simulink library "thermochemical"  (R2017b)
settings: Solver=VariableStepAuto  StartTime=0.0  StopTime=10.0  RelTol=1e-3
values from neighbouring files (symbols this model uses):
  c = conversion_factors()    [blk_clausius_clapeyron.m]    (also in blk_clausius_clapeyron_no_popup.m; blk_cold_room_closed_dry_air.m; blk_reactor_BaCl2_NH3_no_walls.m; blk_reactor_BaCl2_NH3_no_walls_state_space.m)
  cp = metal.cp    [blk_wall_simple.m]    (also in get_metal_properties.m = 390)
  fluid = get_param(blk,'fluid')    [blk_thermodynamic_properties_nonsaturated.m]    (also in blk_thermodynamic_properties_nonsaturated_interpreted.m; blk_thermodynamic_properties_saturated.m; blk_thermodynamic_properties_saturated_interpreted.m; blk_thermodynamic_properties_saturated_mix.m)
  gas = get_material_properties(x.gasName)    [blk_reactor_BaCl2_NH3_cylindrical_no_walls_fun1.m]
  h = get_param(gcb,'ObjectParameters')    [get_param_eval.m]
  rho = metal.rho    [blk_wall_simple.m]    (also in get_metal_properties.m = 8940)
  s = solve(eq,dx,'ReturnConditions',true)    [LMTD_inv.m]    (also in blk_wall_simple.m = get_param_eval(blk,'s'))
  u_gas_at_T_ref = -R * T_ref    [blk_reactor_BaCl2_NH3_no_walls.m]    (also in blk_reactor_BaCl2_NH3_no_walls_state_space.m)
undefined symbols (not defined in the file or in its folder): b_motor, BaCl2, beta, CoolProp, cP_binder, cP_gas, cP_s0, cv, dh_r_0, ENG, heat_exchanger_epsilonNTU_inv_simulink, heat_exchanger_epsilonNTU_simulink, J_motor, K_cin, kappa, Km_motor, La_motor, lookup2D_BreakPoint2, M_binder, N_binder, N_gas_free_volume_init, N_salt, NH3, nh3_v3, nu, P, phase, PID_D_motor, PID_I_motor, PID_P_motor, Ra_motor, Reactor_phase, T, T1, T2, T_init, Tr_init, Tr_ref, U_binder_at_Tr_ref, U_salt_at_X0_Tr_ref, Ur_init, V_void, Valve_regime, Vmax_motor, w_init_motor, X_init
libraries: thermochemical x247, simulink x54, dspsigops x3
(part 4 of 12)

== system thermochemical/Reactors/Reactor, BaCl2//NH3, state-space form, [Tr, Ng, X] as state variables, no algebraic loops, ideal gas in void volume, ideal gas in salt ==
  "Reactor, BaCl2, cylindrical, finned tube, state-space form, [Tr, Ng, X] as state variables, no algebraic loops, ideal gas in void volume" : Subsystem
  "Reactor, BaCl2/NH3, cylindrical, no walls, state-space form, [Tr, Ng, X] as state variables, no algebraic loops, ideal gas in void volume" : Subsystem  LoadFcn=Simulink.defineIntEnumType('Reactor_phase',{'Synthesis','No_reaction','Desorption'},[1 0 -1])  mask(reactor_BaCl2_NH3_cylindrical_no_walls){pairName=Barium chloride/Ammonia (BaCl2/NH3), gasName=Ammonia gas (NH3), binderName=ENG, tao_salt=0.75, rho_composite=300, K_cin=1e-3, fluid=nh3_v3, Lr=1.5, Lr_total=1.6, Dr=0.11, Ddiff=0.018, Tr_init=300, X_init=0.1, Vr_L=15.2053, m_composite_kg=4.162, m_salt_kg=3.1215, m_binder_kg=1.0405, m_gas_when_reactor_fully_charged_kg=2.0423, kWh_cold=0.77838, N_salt=14.9906, N_binder=86.6307, V_void=0.001332, N_gas_free_volume_init=0.16063}
      mask prompts: pairName "Pair name"; gasName "Gas name"; binderName "Binder name"; tao_salt "Salt/Composite mass ratio (mass salt/mass mixture)"; rho_composite "Composite density (kg/m3 of composite)"; K_cin "Reaction's rate constant [1/sec]"; fluid "Gas look-up table data (structure variable):"; Lr "Reactor effective length (section filled with composite) [m]"; Lr_total "Reactor total length ( > effective length) [m]"; Dr "Reactor diameter [m]"; Ddiff "Central diffuser diameter [m]"; Tr_init "Reactor initial temperature [K]"; X_init "Reaction's advancement initial state X0 [0..1]"; Vr_L "Volume reactor (litre)"; m_composite_kg "Mass of composite (salt + binder) (kg)"; m_salt_kg "Mass of salt (kg)"; m_binder_kg "Mass of binder (kg)"; m_gas_when_reactor_fully_charged_kg "Mass of gas (when reactor is fully charged) (kg)"; kWh_cold "Estimated cold production during synthesis (kWh)"; N_salt "Number of mols of salt [mol]"; N_binder "Number of mols of binder [mol]"; V_void "Reactor void volume [m3]"; N_gas_free_volume_init "Initial number of mols of gas in the reactor's free volume [mol]"
      mask help:
      | Solid/Gas thermochemical reactor model, cylindrical shape (no walls)
      | Pair: Barium chloride/Ammonia (BaCl2/NH3)
      mask init:
      | % Note: the enumerated type is declared in 
      | % the 'LoadFnc' callback of the block. In cannot be 
      | % declared here because it gives error for duplicate
      | % declaration.
      | blk_reactor_BaCl2_NH3_cylindrical_no_walls(gcb)
      mask DialogControl Container21 Prompt: Input parameters
      mask DialogControl Container34 Prompt: Reactor's parameters
      mask DialogControl Container31 Prompt: Geometry
      mask DialogControl Container33 Prompt: Reactor Initial state
      mask DialogControl Container18 Prompt: Info (read-only)
      mask DialogControl Container16 Prompt: Base block inputs (read-only)
  "Reactor, BaCl2/NH3, no walls, state-space form, [Tr, Ng, X] as state variables, no algebraic loops, ideal gas in void volume" : Subsystem  LoadFcn=Simulink.defineIntEnumType('Reactor_phase',{'Synthesis','No_reaction','Desorption'},[1 0 -1])  mask(reactor_BaCl2_NH3_no_walls_state_space){pairName=Barium chloride/Ammonia (BaCl2/NH3), gasName=Ammonia gas (NH3), binderName=ENG, N_salt=N_salt, N_binder=N_binder, K_cin=K_cin, V_void=V_void, fluid=fluid, Tr_init=Tr_init, X_init=X_init, N_gas_free_volume_init=N_gas_free_volume_init, m_composite_kg=3.223, m_salt_kg=2.385, m_binder_kg=0.83797, m_gas_when_reactor_fully_charged=1.5605, T_ref=300, u_gas_at_T_ref=0, U_binder_at_T_ref=0, U_salt_at_X0_T_ref=0, R=8.3145, cP_gas=42.5775, cV_gas=29.4370, nu=8, cP_s0=75.1, dh_r_0=38250, M_binder=0.012011, cP_binder=714.36, P_dead_zone=0.0001, dn_dead_zone=0.0001}
      mask prompts: pairName "Pair name"; gasName "Gas name"; binderName "Binder name"; N_salt "Number of mols of salt [mol]"; N_binder "Number of mols of binder [mol]"; K_cin "Reaction's rate constant [1/sec]"; V_void "Reactor void volume [m3]"; fluid "Gas look-up table data (structure variable):"; Tr_init "Reactor initial temperature [K]"; X_init "Reaction's advancement initial state X0 [0..1]"; N_gas_free_volume_init "Initial number of mols of gas in the reactor's void volume [mol]"; m_composite_kg "Mass of composite (salt + binder) (kg)"; m_salt_kg "Mass of salt (kg)"; m_binder_kg "Mass of binder (kg)"; m_gas_when_reactor_fully_charged "Mass of gas (when reactor is fully charged) (kg)"; T_ref "Reference temperature of gas (for the internal energy equation) [K]"; u_gas_at_T_ref "Gas specific internal energy at reference temperature [J/mol]"; U_binder_at_T_ref "Binder internal energy at reference temperature [J]"; U_salt_at_X0_T_ref "Salt internal energy at X=0 and at reference temperature [J]"; R "Universal gas constant [J/K/mol]"; cP_gas "Cp of gas [J/K/mol]"; cV_gas "Cv of gas [J/K/mol]"; nu "Reaction stoichiometric coefficient [mol gas/mol salt]"; cP_s0 "Cp of the anhydrous salt [J/(K.mol)]"; dh_r_0 "Standard enthalpy of reaction [J/mol of gas]"; M_binder "Molar mass of binder [kg/mol]"; cP_binder "Cp of binder [J/(K.kg)]"; P_dead_zone "Presure hystesis to avoid chattering between adsorption and desorption models (typical value: 1e-4) [bar]"; dn_dead_zone "Flow rate hysteresis to avoid chattering between adsorption and desorption models (typical value: 1e-4) [mol/sec]"
      mask help:
      | Solid/Gas thermochemical reactor model (no walls)
      | Pair: Barium chloride/Ammonia (BaCl2/NH3)
      mask init:
      | % Note: the enumerated type is declared in 
      | % the 'LoadFnc' callback of the block. In cannot be 
      | % declared here because it gives error for duplicate
      | % declaration.
      | 
      | blk_reactor_BaCl2_NH3_no_walls_state_space(gcb)
      mask DialogControl Container21 Prompt: Input parameters
      mask DialogControl Container34 Prompt: Reactor's parameters
      mask DialogControl Container33 Prompt: Reactor Initial state
      mask DialogControl Container32 Prompt: Info (read-only)
      mask DialogControl Container16 Prompt: Other read-only parameters
      mask DialogControl Container20 Prompt: References
      mask DialogControl Container18 Prompt: Gas
      mask DialogControl Container47 Prompt: Solid/Gas
      mask DialogControl Container19 Prompt: Binder
      mask DialogControl Container26 Prompt: Other model's parameters

== system thermochemical/Reactors/Reactor, BaCl2//NH3, state-space form, [Tr, Ng, X] as state variables, no algebraic loops, real gas in void volume, ideal gas in salt ==
  "Reactor, BaCl2, cylindrical, finned tube, state-space form, [Tr, Ng, X] as state variables, no algebraic loops, real gas in void volume, ideal gas in salt" : Subsystem
  "Reactor, BaCl2/NH3, cylindrical, no walls, state-space form, [Tr, Ng, X] as state variables, no algebraic loops, real gas in void volume, ideal gas in salt" : Subsystem  LoadFcn=Simulink.defineIntEnumType('Reactor_phase',{'Synthesis','No_reaction','Desorption'},[1 0 -1])  mask(reactor_BaCl2_NH3_cylindrical_no_walls){pairName=Barium chloride/Ammonia (BaCl2/NH3), gasName=Ammonia gas (NH3), binderName=ENG, tao_salt=0.75, rho_composite=300, K_cin=1e-3, fluid=nh3_v3, Lr=1.5, Lr_total=1.6, Dr=0.11, Ddiff=0.018, Tr_init=300, X_init=0.1, Vr_L=15.2053, m_composite_kg=4.162, m_salt_kg=3.1215, m_binder_kg=1.0405, m_gas_when_reactor_fully_charged_kg=2.0423, kWh_cold=0.77838, N_salt=14.9906, N_binder=86.6307, V_void=0.001332, N_gas_free_volume_init=0.16063}
      mask prompts: pairName "Pair name"; gasName "Gas name"; binderName "Binder name"; tao_salt "Salt/Composite mass ratio (mass salt/mass mixture)"; rho_composite "Composite density (kg/m3 of composite)"; K_cin "Reaction's rate constant [1/sec]"; fluid "Gas look-up table data (structure variable):"; Lr "Reactor effective length (section filled with composite) [m]"; Lr_total "Reactor total length ( > effective length) [m]"; Dr "Reactor diameter [m]"; Ddiff "Central diffuser diameter [m]"; Tr_init "Reactor initial temperature [K]"; X_init "Reaction's advancement initial state X0 [0..1]"; Vr_L "Volume reactor (litre)"; m_composite_kg "Mass of composite (salt + binder) (kg)"; m_salt_kg "Mass of salt (kg)"; m_binder_kg "Mass of binder (kg)"; m_gas_when_reactor_fully_charged_kg "Mass of gas (when reactor is fully charged) (kg)"; kWh_cold "Estimated cold production during synthesis (kWh)"; N_salt "Number of mols of salt [mol]"; N_binder "Number of mols of binder [mol]"; V_void "Reactor void volume [m3]"; N_gas_free_volume_init "Initial number of mols of gas in the reactor's free volume [mol]"
      mask help:
      | Solid/Gas thermochemical reactor model, cylindrical shape (no walls)
      | Pair: Barium chloride/Ammonia (BaCl2/NH3)
      mask init: same as thermochemical/Reactors/Reactor, BaCl2//NH3, state-space form, [Tr, Ng, X] as state variables, no algebraic loops, ideal gas in void volume, ideal gas in salt/Reactor, BaCl2/NH3, cylindrical, no walls, state-space form, [Tr, Ng, X] as state variables, no algebraic loops, ideal gas in void volume
      mask DialogControl Container21 Prompt: Input parameters
      mask DialogControl Container34 Prompt: Reactor's parameters
      mask DialogControl Container31 Prompt: Geometry
      mask DialogControl Container33 Prompt: Reactor Initial state
      mask DialogControl Container18 Prompt: Info (read-only)
      mask DialogControl Container16 Prompt: Base block inputs (read-only)
  "Reactor, BaCl2/NH3, no walls, state-space form, [Tr, Ng, X] as state variables, no algebraic loops, real gas in void volume, ideal gas in salt" : Subsystem  LoadFcn=Simulink.defineIntEnumType('Reactor_phase',{'Synthesis','No_reaction','Desorption'},[1 0 -1])  mask(reactor_BaCl2_NH3_no_walls_state_space){pairName=Barium chloride/Ammonia (BaCl2/NH3), gasName=Ammonia gas (NH3), binderName=ENG, N_salt=N_salt, N_binder=N_binder, K_cin=K_cin, V_void=V_void, fluid=fluid, Tr_init=Tr_init, X_init=X_init, N_gas_free_volume_init=N_gas_free_volume_init, m_composite_kg=3.223, m_salt_kg=2.385, m_binder_kg=0.83797, m_gas_when_reactor_fully_charged=1.5605, T_ref=300, u_gas_at_T_ref=0, U_binder_at_T_ref=0, U_salt_at_X0_T_ref=0, R=8.3145, cP_gas=42.5775, cV_gas=29.4370, nu=8, cP_s0=75.1, dh_r_0=38250, M_binder=0.012011, cP_binder=714.36, P_dead_zone=0.0001, dn_dead_zone=0.0001}
      mask prompts: pairName "Pair name"; gasName "Gas name"; binderName "Binder name"; N_salt "Number of mols of salt [mol]"; N_binder "Number of mols of binder [mol]"; K_cin "Reaction's rate constant [1/sec]"; V_void "Reactor void volume [m3]"; fluid "Gas look-up table data (structure variable):"; Tr_init "Reactor initial temperature [K]"; X_init "Reaction's advancement initial state X0 [0..1]"; N_gas_free_volume_init "Initial number of mols of gas in the reactor's void volume [mol]"; m_composite_kg "Mass of composite (salt + binder) (kg)"; m_salt_kg "Mass of salt (kg)"; m_binder_kg "Mass of binder (kg)"; m_gas_when_reactor_fully_charged "Mass of gas (when reactor is fully charged) (kg)"; T_ref "Reference temperature of gas (for the internal energy equation) [K]"; u_gas_at_T_ref "Gas specific internal energy at reference temperature [J/mol]"; U_binder_at_T_ref "Binder internal energy at reference temperature [J]"; U_salt_at_X0_T_ref "Salt internal energy at X=0 and at reference temperature [J]"; R "Universal gas constant [J/K/mol]"; cP_gas "Cp of gas [J/K/mol]"; cV_gas "Cv of gas [J/K/mol]"; nu "Reaction stoichiometric coefficient [mol gas/mol salt]"; cP_s0 "Cp of the anhydrous salt [J/(K.mol)]"; dh_r_0 "Standard enthalpy of reaction [J/mol of gas]"; M_binder "Molar mass of binder [kg/mol]"; cP_binder "Cp of binder [J/(K.kg)]"; P_dead_zone "Presure hystesis to avoid chattering between adsorption and desorption models (typical value: 1e-4) [bar]"; dn_dead_zone "Flow rate hysteresis to avoid chattering between adsorption and desorption models (typical value: 1e-4) [mol/sec]"
      mask help:
      | Solid/Gas thermochemical reactor model (no walls)
      | Pair: Barium chloride/Ammonia (BaCl2/NH3)
      mask init: same as thermochemical/Reactors/Reactor, BaCl2//NH3, state-space form, [Tr, Ng, X] as state variables, no algebraic loops, ideal gas in void volume, ideal gas in salt/Reactor, BaCl2/NH3, no walls, state-space form, [Tr, Ng, X] as state variables, no algebraic loops, ideal gas in void volume
      mask DialogControl Container21 Prompt: Input parameters
      mask DialogControl Container34 Prompt: Reactor's parameters
      mask DialogControl Container33 Prompt: Reactor Initial state
      mask DialogControl Container32 Prompt: Info (read-only)
      mask DialogControl Container16 Prompt: Other read-only parameters
      mask DialogControl Container20 Prompt: References
      mask DialogControl Container18 Prompt: Gas
      mask DialogControl Container47 Prompt: Solid/Gas
      mask DialogControl Container19 Prompt: Binder
      mask DialogControl Container26 Prompt: Other model's parameters

== system thermochemical/Reactors/Reactor, BaCl2//NH3, state-space form, [Tr, Ng, X] as state variables, no algebraic loops, real gas in void volume, real gas in salt ==
  "Reactor, BaCl2, cylindrical, finned tube, state-space form, [Tr, Ng, X] as state variables, no algebraic loops, real gas in void volume, real gas in salt" : Subsystem
  "Reactor, BaCl2/NH3, cylindrical, no walls, state-space form, [Tr, Ng, X] as state variables, no algebraic loops, real gas in void volume, real gas in salt" : Subsystem  LoadFcn=Simulink.defineIntEnumType('Reactor_phase',{'Synthesis','No_reaction','Desorption'},[1 0 -1])  mask(reactor_BaCl2_NH3_cylindrical_no_walls){pairName=Barium chloride/Ammonia (BaCl2/NH3), gasName=Ammonia gas (NH3), binderName=ENG, tao_salt=0.75, rho_composite=300, K_cin=1e-3, fluid=nh3_v3, Lr=1.5, Lr_total=1.6, Dr=0.11, Ddiff=0.018, Tr_init=300, X_init=0.1, Vr_L=15.2053, m_composite_kg=4.162, m_salt_kg=3.1215, m_binder_kg=1.0405, m_gas_when_reactor_fully_charged_kg=2.0423, kWh_cold=0.77838, N_salt=14.9906, N_binder=86.6307, V_void=0.001332, N_gas_free_volume_init=0.16063}
      mask prompts: pairName "Pair name"; gasName "Gas name"; binderName "Binder name"; tao_salt "Salt/Composite mass ratio (mass salt/mass mixture)"; rho_composite "Composite density (kg/m3 of composite)"; K_cin "Reaction's rate constant [1/sec]"; fluid "Gas look-up table data (structure variable):"; Lr "Reactor effective length (section filled with composite) [m]"; Lr_total "Reactor total length ( > effective length) [m]"; Dr "Reactor diameter [m]"; Ddiff "Central diffuser diameter [m]"; Tr_init "Reactor initial temperature [K]"; X_init "Reaction's advancement initial state X0 [0..1]"; Vr_L "Volume reactor (litre)"; m_composite_kg "Mass of composite (salt + binder) (kg)"; m_salt_kg "Mass of salt (kg)"; m_binder_kg "Mass of binder (kg)"; m_gas_when_reactor_fully_charged_kg "Mass of gas (when reactor is fully charged) (kg)"; kWh_cold "Estimated cold production during synthesis (kWh)"; N_salt "Number of mols of salt [mol]"; N_binder "Number of mols of binder [mol]"; V_void "Reactor void volume [m3]"; N_gas_free_volume_init "Initial number of mols of gas in the reactor's free volume [mol]"
      mask help:
      | Solid/Gas thermochemical reactor model, cylindrical shape (no walls)
      | Pair: Barium chloride/Ammonia (BaCl2/NH3)
      mask init: same as thermochemical/Reactors/Reactor, BaCl2//NH3, state-space form, [Tr, Ng, X] as state variables, no algebraic loops, ideal gas in void volume, ideal gas in salt/Reactor, BaCl2/NH3, cylindrical, no walls, state-space form, [Tr, Ng, X] as state variables, no algebraic loops, ideal gas in void volume
      mask DialogControl Container21 Prompt: Input parameters
      mask DialogControl Container34 Prompt: Reactor's parameters
      mask DialogControl Container31 Prompt: Geometry
      mask DialogControl Container33 Prompt: Reactor Initial state
      mask DialogControl Container18 Prompt: Info (read-only)
      mask DialogControl Container16 Prompt: Base block inputs (read-only)
  "Reactor, BaCl2/NH3, no walls, state-space form, [Tr, Ng, X] as state variables, no algebraic loops, real gas in void volume, real gas in salt" : Subsystem  LoadFcn=Simulink.defineIntEnumType('Reactor_phase',{'Synthesis','No_reaction','Desorption'},[1 0 -1])  mask(reactor_BaCl2_NH3_no_walls_state_space){pairName=Barium chloride/Ammonia (BaCl2/NH3), gasName=Ammonia gas (NH3), binderName=ENG, N_salt=N_salt, N_binder=N_binder, K_cin=K_cin, V_void=V_void, fluid=fluid, Tr_init=Tr_init, X_init=X_init, N_gas_free_volume_init=N_gas_free_volume_init, m_composite_kg=3.223, m_salt_kg=2.385, m_binder_kg=0.83797, m_gas_when_reactor_fully_charged=1.5605, T_ref=300, u_gas_at_T_ref=0, U_binder_at_T_ref=0, U_salt_at_X0_T_ref=0, R=8.3145, cP_gas=42.5775, cV_gas=29.4370, nu=8, cP_s0=75.1, dh_r_0=38250, M_binder=0.012011, cP_binder=714.36, P_dead_zone=0.0001, dn_dead_zone=0.0001}
      mask prompts: pairName "Pair name"; gasName "Gas name"; binderName "Binder name"; N_salt "Number of mols of salt [mol]"; N_binder "Number of mols of binder [mol]"; K_cin "Reaction's rate constant [1/sec]"; V_void "Reactor void volume [m3]"; fluid "Gas look-up table data (structure variable):"; Tr_init "Reactor initial temperature [K]"; X_init "Reaction's advancement initial state X0 [0..1]"; N_gas_free_volume_init "Initial number of mols of gas in the reactor's void volume [mol]"; m_composite_kg "Mass of composite (salt + binder) (kg)"; m_salt_kg "Mass of salt (kg)"; m_binder_kg "Mass of binder (kg)"; m_gas_when_reactor_fully_charged "Mass of gas (when reactor is fully charged) (kg)"; T_ref "Reference temperature of gas (for the internal energy equation) [K]"; u_gas_at_T_ref "Gas specific internal energy at reference temperature [J/mol]"; U_binder_at_T_ref "Binder internal energy at reference temperature [J]"; U_salt_at_X0_T_ref "Salt internal energy at X=0 and at reference temperature [J]"; R "Universal gas constant [J/K/mol]"; cP_gas "Cp of gas [J/K/mol]"; cV_gas "Cv of gas [J/K/mol]"; nu "Reaction stoichiometric coefficient [mol gas/mol salt]"; cP_s0 "Cp of the anhydrous salt [J/(K.mol)]"; dh_r_0 "Standard enthalpy of reaction [J/mol of gas]"; M_binder "Molar mass of binder [kg/mol]"; cP_binder "Cp of binder [J/(K.kg)]"; P_dead_zone "Presure hystesis to avoid chattering between adsorption and desorption models (typical value: 1e-4) [bar]"; dn_dead_zone "Flow rate hysteresis to avoid chattering between adsorption and desorption models (typical value: 1e-4) [mol/sec]"
      mask help:
      | Solid/Gas thermochemical reactor model (no walls)
      | Pair: Barium chloride/Ammonia (BaCl2/NH3)
      mask init: same as thermochemical/Reactors/Reactor, BaCl2//NH3, state-space form, [Tr, Ng, X] as state variables, no algebraic loops, ideal gas in void volume, ideal gas in salt/Reactor, BaCl2/NH3, no walls, state-space form, [Tr, Ng, X] as state variables, no algebraic loops, ideal gas in void volume
      mask DialogControl Container21 Prompt: Input parameters
      mask DialogControl Container34 Prompt: Reactor's parameters
      mask DialogControl Container33 Prompt: Reactor Initial state
      mask DialogControl Container32 Prompt: Info (read-only)
      mask DialogControl Container16 Prompt: Other read-only parameters
      mask DialogControl Container20 Prompt: References
      mask DialogControl Container18 Prompt: Gas
      mask DialogControl Container47 Prompt: Solid/Gas
      mask DialogControl Container19 Prompt: Binder
      mask DialogControl Container26 Prompt: Other model's parameters

== system thermochemical/Reactors/Reactor, BaCl2//NH3, state-space form, [Ur, Ng, X] as state variables, no algebraic loops, ideal gas in void volume, ideal gas in salt ==
  "Reactor, BaCl2, cylindrical, finned tube, state-space form, [Ur, Ng, X] as state variables, no algebraic loops, ideal gas in void volume, ideal gas in salt" : Subsystem
  "Reactor, BaCl2/NH3, cylindrical, no walls, state-space form, [Ur, Ng, X] as state variables, no algebraic loops, ideal gas in void volume, ideal gas in salt" : Subsystem  LoadFcn=Simulink.defineIntEnumType('Reactor_phase',{'Synthesis','No_reaction','Desorption'},[1 0 -1])  mask(reactor_BaCl2_NH3_cylindrical_no_walls){pairName=Barium chloride/Ammonia (BaCl2/NH3), gasName=Ammonia gas (NH3), binderName=ENG, tao_salt=0.75, rho_composite=300, K_cin=1e-3, fluid=nh3_v3, Lr=1.5, Lr_total=1.6, Dr=0.11, Ddiff=0.018, Tr_init=300, X_init=0.1, Vr_L=15.2053, m_composite_kg=4.162, m_salt_kg=3.1215, m_binder_kg=1.0405, m_gas_when_reactor_fully_charged_kg=2.0423, kWh_cold=0.77838, N_salt=14.9906, N_binder=86.6307, V_void=0.001332, N_gas_free_volume_init=0.16063}
      mask prompts: pairName "Pair name"; gasName "Gas name"; binderName "Binder name"; tao_salt "Salt/Composite mass ratio (mass salt/mass mixture)"; rho_composite "Composite density (kg/m3 of composite)"; K_cin "Reaction's rate constant [1/sec]"; fluid "Gas look-up table data (structure variable):"; Lr "Reactor effective length (section filled with composite) [m]"; Lr_total "Reactor total length ( > effective length) [m]"; Dr "Reactor diameter [m]"; Ddiff "Central diffuser diameter [m]"; Tr_init "Reactor initial temperature [K]"; X_init "Reaction's advancement initial state X0 [0..1]"; Vr_L "Volume reactor (litre)"; m_composite_kg "Mass of composite (salt + binder) (kg)"; m_salt_kg "Mass of salt (kg)"; m_binder_kg "Mass of binder (kg)"; m_gas_when_reactor_fully_charged_kg "Mass of gas (when reactor is fully charged) (kg)"; kWh_cold "Estimated cold production during synthesis (kWh)"; N_salt "Number of mols of salt [mol]"; N_binder "Number of mols of binder [mol]"; V_void "Reactor void volume [m3]"; N_gas_free_volume_init "Initial number of mols of gas in the reactor's free volume [mol]"
      mask help:
      | Solid/Gas thermochemical reactor model, cylindrical shape (no walls)
      | Pair: Barium chloride/Ammonia (BaCl2/NH3)
      mask init: same as thermochemical/Reactors/Reactor, BaCl2//NH3, state-space form, [Tr, Ng, X] as state variables, no algebraic loops, ideal gas in void volume, ideal gas in salt/Reactor, BaCl2/NH3, cylindrical, no walls, state-space form, [Tr, Ng, X] as state variables, no algebraic loops, ideal gas in void volume
      mask DialogControl Container21 Prompt: Input parameters
      mask DialogControl Container34 Prompt: Reactor's parameters
      mask DialogControl Container31 Prompt: Geometry
      mask DialogControl Container33 Prompt: Reactor Initial state
      mask DialogControl Container18 Prompt: Info (read-only)
      mask DialogControl Container16 Prompt: Base block inputs (read-only)
  "Reactor, BaCl2/NH3, no walls, state-space form, [Ur, Ng, X] as state variables, no algebraic loops, ideal gas in void volume, ideal gas in salt" : Subsystem  LoadFcn=Simulink.defineIntEnumType('Reactor_phase',{'Synthesis','No_reaction','Desorption'},[1 0 -1])  mask(reactor_BaCl2_NH3_no_walls_state_space){pairName=Barium chloride/Ammonia (BaCl2/NH3), gasName=Ammonia gas (NH3), binderName=ENG, N_salt=N_salt, N_binder=N_binder, K_cin=K_cin, V_void=V_void, Tr_init=Tr_init, X_init=X_init, N_gas_free_volume_init=N_gas_free_volume_init, m_composite_kg=4.1639, m_salt_kg=3.1235, m_binder_kg=1.0405, m_gas_when_reactor_fully_charged=2.0436, T_ref=300, u_gas_at_T_ref=0, U_binder_at_T_ref=0, U_salt_at_X0_T_ref=0, R=8.3145, cP_gas=42.5775, nu=8, cP_s0=75.1, dh_r_0=38250, M_binder=0.012011, cP_binder=714.36, P_dead_zone=0.0001, dn_dead_zone=0.0001}
      mask prompts: pairName "Pair name"; gasName "Gas name"; binderName "Binder name"; N_salt "Number of mols of salt [mol]"; N_binder "Number of mols of binder [mol]"; K_cin "Reaction's rate constant [1/sec]"; V_void "Reactor void volume [m3]"; Tr_init "Reactor initial temperature [K]"; X_init "Reaction's advancement initial state X0 [0..1]"; N_gas_free_volume_init "Initial number of mols of gas in the reactor's void volume [mol]"; m_composite_kg "Mass of composite (salt + binder) (kg)"; m_salt_kg "Mass of salt (kg)"; m_binder_kg "Mass of binder (kg)"; m_gas_when_reactor_fully_charged "Mass of gas (when reactor is fully charged) (kg)"; T_ref "Reference temperature of gas (for the internal energy equation) [K]"; u_gas_at_T_ref "Gas specific internal energy at reference temperature [J/mol]"; U_binder_at_T_ref "Binder internal energy at reference temperature [J]"; U_salt_at_X0_T_ref "Salt internal energy at X=0 and at reference temperature [J]"; R "Universal gas constant [J/K/mol]"; cP_gas "Cp of gas [J/K/mol]"; nu "Reaction stoichiometric coefficient [mol gas/mol salt]"; cP_s0 "Cp of the anhydrous salt [J/(K.mol)]"; dh_r_0 "Standard enthalpy of reaction [J/mol of gas]"; M_binder "Molar mass of binder [kg/mol]"; cP_binder "Cp of binder [J/(K.kg)]"; P_dead_zone "Presure hystesis to avoid chattering between adsorption and desorption models (typical value: 1e-4) [bar]"; dn_dead_zone "Flow rate hysteresis to avoid chattering between adsorption and desorption models (typical value: 1e-4) [mol/sec]"
      mask help:
      | Solid/Gas thermochemical reactor model (no walls)
      | Pair: Barium chloride/Ammonia (BaCl2/NH3)
      mask init: same as thermochemical/Reactors/Reactor, BaCl2//NH3, state-space form, [Tr, Ng, X] as state variables, no algebraic loops, ideal gas in void volume, ideal gas in salt/Reactor, BaCl2/NH3, no walls, state-space form, [Tr, Ng, X] as state variables, no algebraic loops, ideal gas in void volume
      mask DialogControl Container21 Prompt: Input parameters
      mask DialogControl Container34 Prompt: Reactor's parameters
      mask DialogControl Container33 Prompt: Reactor Initial state
      mask DialogControl Container32 Prompt: Info (read-only)
      mask DialogControl Container16 Prompt: Other read-only parameters
      mask DialogControl Container18_copy Prompt: References
      mask DialogControl Container18 Prompt: Gas
      mask DialogControl Container47 Prompt: Solid/Gas
      mask DialogControl Container19 Prompt: Binder
      mask DialogControl Container26 Prompt: Other model's parameters

== system thermochemical/Reactors/Reactor, BaCl2//NH3, with algebraic loops, ideal gas in void volume, ideal gas in salt ==
  "Reactor, BaCl2, cylindrical, finned tube, with algebraic loops, ideal gas in void volume, ideal gas in salt" : Subsystem
  "Reactor, BaCl2/NH3, cylindrical, no walls, with algebraic loops, ideal gas in void volume, ideal gas in salt" : Subsystem  LoadFcn=Simulink.defineIntEnumType('Reactor_phase',{'Synthesis','No_reaction','Desorption'},[1 0 -1])  mask(reactor_BaCl2_NH3_cylindrical_no_walls){pairName=Barium chloride/Ammonia (BaCl2/NH3), gasName=Ammonia gas (NH3), binderName=ENG, tao_salt=0.75, rho_composite=300, K_cin=1e-3, fluid=nh3_v3, Lr=1.5, Lr_total=1.6, Dr=0.11, Ddiff=0.018, Tr_init=300, X_init=0.1, Vr_L=15.2053, m_composite_kg=4.162, m_salt_kg=3.1215, m_binder_kg=1.0405, m_gas_when_reactor_fully_charged_kg=2.0423, kWh_cold=0.77838, N_salt=14.9906, N_binder=86.6307, V_void=0.001332, N_gas_free_volume_init=0.16063}
      mask prompts: pairName "Pair name"; gasName "Gas name"; binderName "Binder name"; tao_salt "Salt/Composite mass ratio (mass salt/mass mixture)"; rho_composite "Composite density (kg/m3 of composite)"; K_cin "Reaction's rate constant [1/sec]"; fluid "Gas look-up table data (structure variable):"; Lr "Reactor effective length (section filled with composite) [m]"; Lr_total "Reactor total length ( > effective length) [m]"; Dr "Reactor diameter [m]"; Ddiff "Central diffuser diameter [m]"; Tr_init "Reactor initial temperature [K]"; X_init "Reaction's advancement initial state X0 [0..1]"; Vr_L "Volume reactor (litre)"; m_composite_kg "Mass of composite (salt + binder) (kg)"; m_salt_kg "Mass of salt (kg)"; m_binder_kg "Mass of binder (kg)"; m_gas_when_reactor_fully_charged_kg "Mass of gas (when reactor is fully charged) (kg)"; kWh_cold "Estimated cold production during synthesis (kWh)"; N_salt "Number of mols of salt [mol]"; N_binder "Number of mols of binder [mol]"; V_void "Reactor void volume [m3]"; N_gas_free_volume_init "Initial number of mols of gas in the reactor's free volume [mol]"
      mask help:
      | Solid/Gas thermochemical reactor model, cylindrical shape (no walls)
      | Pair: Barium chloride/Ammonia (BaCl2/NH3)
      mask init: same as thermochemical/Reactors/Reactor, BaCl2//NH3, state-space form, [Tr, Ng, X] as state variables, no algebraic loops, ideal gas in void volume, ideal gas in salt/Reactor, BaCl2/NH3, cylindrical, no walls, state-space form, [Tr, Ng, X] as state variables, no algebraic loops, ideal gas in void volume
      mask DialogControl Container21 Prompt: Input parameters
      mask DialogControl Container34 Prompt: Reactor's parameters
      mask DialogControl Container31 Prompt: Geometry
      mask DialogControl Container33 Prompt: Reactor Initial state
      mask DialogControl Container18 Prompt: Info (read-only)
      mask DialogControl Container16 Prompt: Base block inputs (read-only)
  "Reactor, BaCl2/NH3, no walls, with algebraic loops, ideal gas in void volume, ideal gas in salt" : Subsystem  LoadFcn=Simulink.defineIntEnumType('Reactor_phase',{'Synthesis','No_reaction','Desorption'},[1 0 -1])  mask(reactor_BaCl2_NH3_no_walls){pairName=Barium chloride/Ammonia (BaCl2/NH3), gasName=Ammonia gas (NH3), binderName=ENG, N_salt=N_salt, N_binder=N_binder, K_cin=K_cin, V_void=V_void, fluid=fluid, Tr_init=Tr_init, X_init=X_init, N_gas_free_volume_init=N_gas_free_volume_init, m_composite_kg=, m_salt_kg=, m_binder_kg=, m_gas_when_reactor_fully_charged=, T_ref=239.8236, u_gas_at_T_ref=-1994.0066, U_binder_at_T_ref=0, U_salt_at_X0_T_ref=0, cP_gas=42.5775, nu=8, cP_s0=75.1, Pr_0=1e-05, dh_r_0=38250, ds_r_0=232.38, M_binder=0.012011, cP_binder=714.36, P_dead_zone=0.0001, dn_dead_zone=0.0001, R=8.3145}
      mask prompts: pairName "Pair name"; gasName "Gas name"; binderName "Binder name"; N_salt "Number of mols of salt [mol]"; N_binder "Number of mols of binder [mol]"; K_cin "Reaction's rate constant [1/sec]"; V_void "Reactor void volume [m3]"; fluid "Gas look-up table data (structure variable):"; Tr_init "Reactor initial temperature [K]"; X_init "Reaction's advancement initial state X0 [0..1]"; N_gas_free_volume_init "Initial number of mols of gas in the reactor's void volume [mol]"; m_composite_kg "Mass of composite (salt + binder) (kg)"; m_salt_kg "Mass of salt (kg)"; m_binder_kg "Mass of binder (kg)"; m_gas_when_reactor_fully_charged "Mass of gas (when reactor is fully charged) (kg)"; T_ref "Reference temperature (for the internal energy equations) [K]"; u_gas_at_T_ref "Gas specific internal energy at reference temperature (when ideal gas model is selected) [J/mol]"; U_binder_at_T_ref "Binder internal energy at reference temperature [J]"; U_salt_at_X0_T_ref "Salt internal energy at X=0 and at reference temperature [J]"; cP_gas "and in the reactor's internal energy equation [J/K/mol]"; nu "Reaction stoichiometric coefficient [mol gas/mol salt]"; cP_s0 "Cp of the anhydrous salt [J/(K.mol)]"; Pr_0 "P-T curve, reference pressure P0 [bar]"; dh_r_0 "P-T curve, reference enthalpy dh0 [J/mol]"; ds_r_0 "P-T curve, reference entropy ds0 [J/mol/K]"; M_binder "Molar mass of binder [kg/mol]"; cP_binder "Cp of binder [J/(K.kg)]"; P_dead_zone "Presure hysteresis to avoid chattering between adsorption and desorption models (typical value: 1e-4) [bar]"; dn_dead_zone "Flow rate hysteresis to avoid chattering between adsorption and desorption models (typical value: 1e-4) [mol/sec]"; R "Universal gas constant [J/K/mol]"
      mask help:
      | Solid/Gas thermochemical reactor model (no walls)
      | Pair: Barium chloride/Ammonia (BaCl2/NH3)
      mask init:
      | % Note: the enumerated type is declared in 
      | % the 'LoadFnc' callback of the block. In cannot be 
      | % declared here because it gives error for duplicate
      | % declaration.
      | 
      | blk_reactor_BaCl2_NH3_no_walls(gcb)
      mask DialogControl Container21 Prompt: Input parameters
      mask DialogControl Container34 Prompt: Reactor's parameters
      mask DialogControl Container33 Prompt: Reactor Initial state
      mask DialogControl Container32 Prompt: Info (read-only)
      mask DialogControl Container16 Prompt: Other read-only parameters
      mask DialogControl Container18_copy Prompt: References
      mask DialogControl Control3 Prompt: NOTE: when a real-gas model is selected, the gas specific internal energy at reference temperature is fixed by the gas pre-computed structure variable.
      mask DialogControl Container18 Prompt: Gas
      mask DialogControl Control5 Prompt: cP of gas, used in the reactor's void volume (if ideal model is selected)
      mask DialogControl Container47 Prompt: Solid/Gas
      mask DialogControl Control17 Prompt: Solid/gas: reactor's Clapeyron P-T curve:
      mask DialogControl Container19 Prompt: Binder
      mask DialogControl Container26 Prompt: Other model's parameters
      mask DialogControl Container43 Prompt: General parameters

== system thermochemical/Reactors/Reactor, BaCl2//NH3, with algebraic loops, real gas in void volume, ideal gas in salt ==
  "Reactor, BaCl2/NH3, cylindrical, finned tube, with algebraic loops, real gas in void volume, ideal gas in salt" : Subsystem
  "Reactor, BaCl2/NH3, cylindrical, no walls, with algebraic loops, real gas in void volume, ideal gas in salt" : Subsystem  LoadFcn=Simulink.defineIntEnumType('Reactor_phase',{'Synthesis','No_reaction','Desorption'},[1 0 -1])  mask(reactor_BaCl2_NH3_cylindrical_no_walls){pairName=Barium chloride/Ammonia (BaCl2/NH3), gasName=Ammonia gas (NH3), binderName=ENG, tao_salt=0.75, rho_composite=300, K_cin=1e-3, fluid=nh3_v3, Lr=1.5, Lr_total=1.6, Dr=0.11, Ddiff=0.018, Tr_init=300, X_init=0.1, Vr_L=15.2053, m_composite_kg=4.162, m_salt_kg=3.1215, m_binder_kg=1.0405, m_gas_when_reactor_fully_charged_kg=2.0423, kWh_cold=0.77838, N_salt=14.9906, N_binder=86.6307, V_void=0.001332, N_gas_free_volume_init=0.16063}
      mask prompts: pairName "Pair name"; gasName "Gas name"; binderName "Binder name"; tao_salt "Salt/Composite mass ratio (mass salt/mass mixture)"; rho_composite "Composite density (kg/m3 of composite)"; K_cin "Reaction's rate constant [1/sec]"; fluid "Gas look-up table data (structure variable):"; Lr "Reactor effective length (section filled with composite) [m]"; Lr_total "Reactor total length ( > effective length) [m]"; Dr "Reactor diameter [m]"; Ddiff "Central diffuser diameter [m]"; Tr_init "Reactor initial temperature [K]"; X_init "Reaction's advancement initial state X0 [0..1]"; Vr_L "Volume reactor (litre)"; m_composite_kg "Mass of composite (salt + binder) (kg)"; m_salt_kg "Mass of salt (kg)"; m_binder_kg "Mass of binder (kg)"; m_gas_when_reactor_fully_charged_kg "Mass of gas (when reactor is fully charged) (kg)"; kWh_cold "Estimated cold production during synthesis (kWh)"; N_salt "Number of mols of salt [mol]"; N_binder "Number of mols of binder [mol]"; V_void "Reactor void volume [m3]"; N_gas_free_volume_init "Initial number of mols of gas in the reactor's free volume [mol]"
      mask help:
      | Solid/Gas thermochemical reactor model, cylindrical shape (no walls)
      | Pair: Barium chloride/Ammonia (BaCl2/NH3)
      mask init: same as thermochemical/Reactors/Reactor, BaCl2//NH3, state-space form, [Tr, Ng, X] as state variables, no algebraic loops, ideal gas in void volume, ideal gas in salt/Reactor, BaCl2/NH3, cylindrical, no walls, state-space form, [Tr, Ng, X] as state variables, no algebraic loops, ideal gas in void volume
      mask DialogControl Container21 Prompt: Input parameters
      mask DialogControl Container34 Prompt: Reactor's parameters
      mask DialogControl Container31 Prompt: Geometry
      mask DialogControl Container33 Prompt: Reactor Initial state
      mask DialogControl Container18 Prompt: Info (read-only)
      mask DialogControl Container16 Prompt: Base block inputs (read-only)
  "Reactor, BaCl2/NH3, no walls, with algebraic loops, real gas in void volume, ideal gas in salt" : Subsystem  LoadFcn=Simulink.defineIntEnumType('Reactor_phase',{'Synthesis','No_reaction','Desorption'},[1 0 -1])  mask(reactor_BaCl2_NH3_no_walls){pairName=Barium chloride/Ammonia (BaCl2/NH3), gasName=Ammonia gas (NH3), binderName=ENG, N_salt=N_salt, N_binder=N_binder, K_cin=K_cin, V_void=V_void, fluid=fluid, Tr_init=Tr_init, X_init=X_init, N_gas_free_volume_init=N_gas_free_volume_init, m_composite_kg=4.1639, m_salt_kg=3.1235, m_binder_kg=1.0405, m_gas_when_reactor_fully_charged=2.0436, T_ref=300, u_gas_at_T_ref=0, U_binder_at_T_ref=0, U_salt_at_X0_T_ref=0, cP_gas=42.5775, nu=8, cP_s0=75.1, Pr_0=1e-05, dh_r_0=38250, ds_r_0=232.38, M_binder=0.012011, cP_binder=714.36, P_dead_zone=0.0001, dn_dead_zone=0.0001, R=8.3145}
      mask prompts: pairName "Pair name"; gasName "Gas name"; binderName "Binder name"; N_salt "Number of mols of salt [mol]"; N_binder "Number of mols of binder [mol]"; K_cin "Reaction's rate constant [1/sec]"; V_void "Reactor void volume [m3]"; fluid "Gas look-up table data (structure variable):"; Tr_init "Reactor initial temperature [K]"; X_init "Reaction's advancement initial state X0 [0..1]"; N_gas_free_volume_init "Initial number of mols of gas in the reactor's void volume [mol]"; m_composite_kg "Mass of composite (salt + binder) (kg)"; m_salt_kg "Mass of salt (kg)"; m_binder_kg "Mass of binder (kg)"; m_gas_when_reactor_fully_charged "Mass of gas (when reactor is fully charged) (kg)"; T_ref "Reference temperature of gas (for the internal energy equation) [K]"; u_gas_at_T_ref "Gas specific internal energy at reference temperature (for ideal gas models only) [J/mol]"; U_binder_at_T_ref "Binder internal energy at reference temperature [J]"; U_salt_at_X0_T_ref "Salt internal energy at X=0 and at reference temperature [J]"; cP_gas "cP of gas, used in the reactor's void volume (superheated) [J/K/mol]"; nu "Reaction stoichiometric coefficient [mol gas/mol salt]"; cP_s0 "Cp of the anhydrous salt [J/(K.mol)]"; Pr_0 "P-T curve, reference pressure P0 [bar]"; dh_r_0 "P-T curve, reference enthalpy dh0 [J/mol]"; ds_r_0 "P-T curve, reference entropy ds0 [J/mol/K]"; M_binder "Molar mass of binder [kg/mol]"; cP_binder "Cp of binder [J/(K.kg)]"; P_dead_zone "Presure hystesis to avoid chattering between adsorption and desorption models (typical value: 1e-4) [bar]"; dn_dead_zone "Flow rate hysteresis to avoid chattering between adsorption and desorption models (typical value: 1e-4) [mol/sec]"; R "Universal gas constant [J/K/mol]"
      mask help:
      | Solid/Gas thermochemical reactor model (no walls)
      | Pair: Barium chloride/Ammonia (BaCl2/NH3)
      mask init: same as thermochemical/Reactors/Reactor, BaCl2//NH3, with algebraic loops, ideal gas in void volume, ideal gas in salt/Reactor, BaCl2/NH3, no walls, with algebraic loops, ideal gas in void volume, ideal gas in salt
      mask DialogControl Container21 Prompt: Input parameters
      mask DialogControl Container34 Prompt: Reactor's parameters
      mask DialogControl Container33 Prompt: Reactor Initial state
      mask DialogControl Container32 Prompt: Info (read-only)
      mask DialogControl Container16 Prompt: Other read-only parameters
      mask DialogControl Container18_copy Prompt: References
      mask DialogControl Control3 Prompt: NOTE: For the real gas model, the gas specific internal energy at reference temperature is fixed by the gas look-up table (structure variable).
      mask DialogControl Container18 Prompt: Gas
      mask DialogControl Container47 Prompt: Solid/Gas
      mask DialogControl Control17 Prompt: Solid/gas: reactor's Clapeyron P-T curve:
      mask DialogControl Container19 Prompt: Binder
      mask DialogControl Container26 Prompt: Other model's parameters
      mask DialogControl Container43 Prompt: General parameters

== system thermochemical/Reactors/Reactor, BaCl2//NH3, with algebraic loops, real gas in void volume, real gas in salt ==
  "Reactor, BaCl2, cylindrical, finned tube, with algebraic loops, real gas in void volume, real gas in salt" : Subsystem
  "Reactor, BaCl2/NH3, cylindrical, no walls, with algebraic loops, real gas in void volume, real gas in salt" : Subsystem  LoadFcn=Simulink.defineIntEnumType('Reactor_phase',{'Synthesis','No_reaction','Desorption'},[1 0 -1])  mask(reactor_BaCl2_NH3_cylindrical_no_walls){pairName=Barium chloride/Ammonia (BaCl2/NH3), gasName=Ammonia gas (NH3), binderName=ENG, tao_salt=0.75, rho_composite=300, K_cin=1e-3, fluid=nh3_v3, Lr=1.5, Lr_total=1.6, Dr=0.11, Ddiff=0.018, Tr_init=300, X_init=0.1, Vr_L=15.2053, m_composite_kg=4.162, m_salt_kg=3.1215, m_binder_kg=1.0405, m_gas_when_reactor_fully_charged_kg=2.0423, kWh_cold=0.77838, N_salt=14.9906, N_binder=86.6307, V_void=0.001332, N_gas_free_volume_init=0.16063}
      mask prompts: pairName "Pair name"; gasName "Gas name"; binderName "Binder name"; tao_salt "Salt/Composite mass ratio (mass salt/mass mixture)"; rho_composite "Composite density (kg/m3 of composite)"; K_cin "Reaction's rate constant [1/sec]"; fluid "Gas look-up table data (structure variable):"; Lr "Reactor effective length (section filled with composite) [m]"; Lr_total "Reactor total length ( > effective length) [m]"; Dr "Reactor diameter [m]"; Ddiff "Central diffuser diameter [m]"; Tr_init "Reactor initial temperature [K]"; X_init "Reaction's advancement initial state X0 [0..1]"; Vr_L "Volume reactor (litre)"; m_composite_kg "Mass of composite (salt + binder) (kg)"; m_salt_kg "Mass of salt (kg)"; m_binder_kg "Mass of binder (kg)"; m_gas_when_reactor_fully_charged_kg "Mass of gas (when reactor is fully charged) (kg)"; kWh_cold "Estimated cold production during synthesis (kWh)"; N_salt "Number of mols of salt [mol]"; N_binder "Number of mols of binder [mol]"; V_void "Reactor void volume [m3]"; N_gas_free_volume_init "Initial number of mols of gas in the reactor's free volume [mol]"
      mask help:
      | Solid/Gas thermochemical reactor model, cylindrical shape (no walls)
      | Pair: Barium chloride/Ammonia (BaCl2/NH3)
      mask init: same as thermochemical/Reactors/Reactor, BaCl2//NH3, state-space form, [Tr, Ng, X] as state variables, no algebraic loops, ideal gas in void volume, ideal gas in salt/Reactor, BaCl2/NH3, cylindrical, no walls, state-space form, [Tr, Ng, X] as state variables, no algebraic loops, ideal gas in void volume
      mask DialogControl Container21 Prompt: Input parameters
      mask DialogControl Container34 Prompt: Reactor's parameters
      mask DialogControl Container31 Prompt: Geometry
      mask DialogControl Container33 Prompt: Reactor Initial state
      mask DialogControl Container18 Prompt: Info (read-only)
      mask DialogControl Container16 Prompt: Base block inputs (read-only)
  "Reactor, BaCl2/NH3, no walls, with algebraic loops, real gas in void volume, real gas in salt" : Subsystem  LoadFcn=Simulink.defineIntEnumType('Reactor_phase',{'Synthesis','No_reaction','Desorption'},[1 0 -1])  mask(reactor_BaCl2_NH3_no_walls){pairName=Barium chloride/Ammonia (BaCl2/NH3), gasName=Ammonia gas (NH3), binderName=ENG, N_salt=N_salt, N_binder=N_binder, K_cin=K_cin, V_void=V_void, fluid=fluid, Tr_init=Tr_init, X_init=X_init, N_gas_free_volume_init=N_gas_free_volume_init, m_composite_kg=4.1639, m_salt_kg=3.1235, m_binder_kg=1.0405, m_gas_when_reactor_fully_charged=2.0436, T_ref=300, u_gas_at_T_ref=0, U_binder_at_T_ref=0, U_salt_at_X0_T_ref=0, cP_gas=42.5775, nu=8, cP_s0=75.1, Pr_0=1e-05, dh_r_0=38250, ds_r_0=232.38, M_binder=0.012011, cP_binder=714.36, P_dead_zone=0.0001, dn_dead_zone=0.0001, R=8.3145}
      mask prompts: pairName "Pair name"; gasName "Gas name"; binderName "Binder name"; N_salt "Number of mols of salt [mol]"; N_binder "Number of mols of binder [mol]"; K_cin "Reaction's rate constant [1/sec]"; V_void "Reactor void volume [m3]"; fluid "Gas look-up table data (structure variable):"; Tr_init "Reactor initial temperature [K]"; X_init "Reaction's advancement initial state X0 [0..1]"; N_gas_free_volume_init "Initial number of mols of gas in the reactor's void volume [mol]"; m_composite_kg "Mass of composite (salt + binder) (kg)"; m_salt_kg "Mass of salt (kg)"; m_binder_kg "Mass of binder (kg)"; m_gas_when_reactor_fully_charged "Mass of gas (when reactor is fully charged) (kg)"; T_ref "Reference temperature of gas (for the internal energy equation) [K]"; u_gas_at_T_ref "Gas specific internal energy at reference temperature (for ideal gas models only) [J/mol]"; U_binder_at_T_ref "Binder internal energy at reference temperature [J]"; U_salt_at_X0_T_ref "Salt internal energy at X=0 and at reference temperature [J]"; cP_gas "cP of gas, used in the reactor's void volume (superheated) [J/K/mol]"; nu "Reaction stoichiometric coefficient [mol gas/mol salt]"; cP_s0 "Cp of the anhydrous salt [J/(K.mol)]"; Pr_0 "P-T curve, reference pressure P0 [bar]"; dh_r_0 "P-T curve, reference enthalpy dh0 [J/mol]"; ds_r_0 "P-T curve, reference entropy ds0 [J/mol/K]"; M_binder "Molar mass of binder [kg/mol]"; cP_binder "Cp of binder [J/(K.kg)]"; P_dead_zone "Presure hystesis to avoid chattering between adsorption and desorption models (typical value: 1e-4) [bar]"; dn_dead_zone "Flow rate hysteresis to avoid chattering between adsorption and desorption models (typical value: 1e-4) [mol/sec]"; R "Universal gas constant [J/K/mol]"
      mask help:
      | Solid/Gas thermochemical reactor model (no walls)
      | Pair: Barium chloride/Ammonia (BaCl2/NH3)
      mask init: same as thermochemical/Reactors/Reactor, BaCl2//NH3, with algebraic loops, ideal gas in void volume, ideal gas in salt/Reactor, BaCl2/NH3, no walls, with algebraic loops, ideal gas in void volume, ideal gas in salt
      mask DialogControl Container21 Prompt: Input parameters
      mask DialogControl Container34 Prompt: Reactor's parameters
      mask DialogControl Container33 Prompt: Reactor Initial state
      mask DialogControl Container32 Prompt: Info (read-only)
      mask DialogControl Container16 Prompt: Other read-only parameters
      mask DialogControl Container18_copy Prompt: References
      mask DialogControl Control3 Prompt: NOTE: For the real gas model, the gas specific internal energy at reference temperature is fixed by the gas look-up table (structure variable).
      mask DialogControl Container18 Prompt: Gas
      mask DialogControl Container47 Prompt: Solid/Gas
      mask DialogControl Control17 Prompt: Solid/gas: reactor's Clapeyron P-T curve:
      mask DialogControl Container19 Prompt: Binder
      mask DialogControl Container26 Prompt: Other model's parameters
      mask DialogControl Container43 Prompt: General parameters

== system thermochemical/Thermal loads/Cold room, closed, dry air (it uses CoolProp library for initialization) ==
  In5 : Inport
  In1 : Inport  Port=2
  In8 : Inport  Port=3
  Constant : Constant  Value=[S;V;M;Cv]
  Display4 : Display
  Gain : Gain  Gain=U
  Gain1 : Gain  Gain=S
  Gain12 : Gain  Gain=1/(M*Cv)
  Integrator : Integrator  InitialCondition=Tinit_C
  Sum : Sum  Inputs=|+-
  Sum2 : Sum  Inputs=-++
  Out3 : Outport
  wires:
  Gain12/1 -> Integrator/1  "dTroom/dt"
  Sum2/1 -> Gain12/1  "q net (W)"
  Gain1/1 -> Sum2/3  "q exterior→room (W)"
  Gain/1 -> Gain1/1
  Sum/1 -> Gain/1
  In8/1 -> Sum2/1  "q room→evaporator wall (W)"
  In1/1 -> Sum/1  "T ext (°C)"
  Integrator/1 -> Out3/1, Sum/2  "T room (°C)"
  In5/1 -> Sum2/2  "Heat load (W) (fans, lighting, etc)"
  Constant/1 -> Display4/1

== system thermochemical/Thermodynamic fluid properties/Clausius-Clapeyron ==
  In1 : Inport
  Fcn : Fcn  Expr=1e-05 * exp(-4600.4124/u(1) + 27.9489)
  Out1 : Outport
  wires:
  In1/1 -> Fcn/1  "(K)"
  Fcn/1 -> Out1/1  "(bar)"
